simulink model "TestBenchModel"  (R2019b)
settings: Solver=VariableStepAuto  StartTime=0.0  StopTime=60  FixedStep=0.0001  RelTol=1e-3  EnableMultiTasking=on
InitFcn:
  | TestBenchData;
StartFcn:
  | TestBenchData;
values from neighbouring files (symbols this model uses):
  C = 0.0056    [TestBenchData.m]
  C1 = C    (= 0.0056)    [TestBenchData.m]
  C2 = C1    (= 0.0056)    [TestBenchData.m]
  C3 = C1    (= 0.0056)    [TestBenchData.m]
  C4 = C1    (= 0.0056)    [TestBenchData.m]
  C5 = C1    (= 0.0056)    [TestBenchData.m]
  C6 = C1    (= 0.0056)    [TestBenchData.m]
  Cfc = 0.35    [TestBenchData.m]
  Fs = 1000    [TestBenchData.m]
  glg = 4    [TestBenchData.m]
  gug = 3    [TestBenchData.m]
  Ic1 = 0.05*10^(-3)    (= 5e-05)    [TestBenchData.m]
  Ic4 = Ic3    (= 0.00012)    [TestBenchData.m]
  Ic_mf = 1.1420e-04    (= 0.0001142)    [TestBenchData.m]
  Ifc_1 = 0.003*10^(-3)    (= 3e-06)    [TestBenchData.m]
  Ifc_2 = 0.003*10^(-3)    (= 3e-06)    [TestBenchData.m]
  Imotor = 0.00068    [TestBenchData.m]
  Iprop = gml^2*I_ML + I_GL + Iprop0    [TestBenchData.m]
  Kc1 = 41.9*10^3    (= 41900)    [TestBenchData.m]
  Kc2 = Kc1    (= 41900)    [TestBenchData.m]
  Kc3 = 31*10^3    (= 31000)    [TestBenchData.m]
  Kc4 = Kc3    (= 31000)    [TestBenchData.m]
  Kc5 = 138*10^3    (= 138000)    [TestBenchData.m]
  Kc6 = Kc5    (= 138000)    [TestBenchData.m]
  Kc_mf = 1.9039e+05    (= 190390)    [TestBenchData.m]
  Kfc = 90    [TestBenchData.m]
  Klg = 44.3*10^3    (= 44300)    [TestBenchData.m]
  Km1 = 5.4*10^3    (= 5400)    [TestBenchData.m]
  Km2 = 20*10^3    (= 20000)    [TestBenchData.m]
  Kug = 43.3*10^3    (= 43300)    [TestBenchData.m]
  lg = C1    (= 0.0056)    [TestBenchData.m]
  M1 = S1    (= 0.0056)    [TestBenchData.m]
  M2 = M1    (= 0.0056)    [TestBenchData.m]
  n = 3221    [TestBenchData.m]
  n_idle = 0    [TestBenchData.m]
  Nmill = 12    [TestBenchData.m]
  P = 1150    [TestBenchData.m]
  prop_blades = 4    [TestBenchData.m]
  S = 0.0056    [TestBenchData.m]
  S1 = S    (= 0.0056)    [TestBenchData.m]
  S2 = S1    (= 0.0056)    [TestBenchData.m]
  S3 = S1    (= 0.0056)    [TestBenchData.m]
  S4 = S1    (= 0.0056)    [TestBenchData.m]
  S5 = S1    (= 0.0056)    [TestBenchData.m]
  T = P/(n/9.55)    (= 3.40965538653)    [TestBenchData.m]
  Tice = 100000    [TestBenchData.m]
  To = 0.2    [TestBenchData.m]
  Todelta = 0.5    [TestBenchData.m]
  ug = C1    (= 0.0056)    [TestBenchData.m]
  W = 131.9469    [TestBenchData.m]
  x4 = 0.06/4    (= 0.015)    [TestBenchData.m]
  x8 = 0.02/4    (= 0.005)    [TestBenchData.m]
  Z = 4    [TestBenchData.m]
  z1 = 17    [TestBenchData.m]
  z2 = 42    [TestBenchData.m]
undefined symbols (not defined in the file or in its folder): C1_22, C1_3, C_crank, C_cyl, Data, Iem, Is1, Is2, Is3, Is4, Is5, K1_11, K1_13, K1_15, K1_21, K1_23, K1_5, K1_7, K1_9, Ks1, Ks2, Ks3, Ks4, Ks5, Ks_mf, RPM, Tu
libraries: fl_lib x201, nesl_utility x92, simulink x22, dspstat3 x1
(part 1 of 3)
settings Model: Creator=jupo  LastModifiedBy=Mikael
settings DataIOCC: LimitDataPoints=on  SaveFormat=Array  SignalLoggingSaveFormat=ModelDataLogs  ReturnWorkspaceOutputs=off
settings OptimizationCC: BlockReduction=off  DefaultParameterBehavior=Inlined  BufferReuse=off  ExpressionDepthLimit=2147483647  LifeSpan=inf
settings DebuggingCC: UnderspecifiedInitializationDetection=Classic  MergeDetectMultiDrivingBlocksExec=none  SolverPrmCheckMsg=warning  FcnCallInpInsideContextMsg=warning  StateNameClashWarn=warning  SFUnexpectedBacktrackingDiag=warning  SFNoUnconditionalDefaultTransitionDiag=warning  ArithmeticOperatorsInVariantConditions=warning
settings HardwareCC: ProdBitPerPointer=32  ProdBitPerSizeT=32  ProdBitPerPtrDiffT=32  ProdLargestAtomicFloat=None  ProdWordSize=32  ProdHWDeviceType=Intel->x86/Pentium
settings ModelReferenceCC: EnableParallelModelReferenceBuilds=on  PropagateSignalLabelsOutOfModel=off
settings SFSimCC: SimUseLocalCustomCode=off  CustomCodeUndefinedFunction=UseInterfaceOnly
settings RTWCC: RTWUseLocalCustomCode=off
settings CodeAppCC: StateflowObjectComments=on
settings GRTTargetCC: TargetLangStandard=C89/C90 (ANSI)  GeneratePreprocessorConditionals=Disable all  CombineOutputUpdateFcns=off  GRTInterface=on
settings ConfigComp: CovMetricSettings=dw  CovHtmlReporting=on  CovSaveCumulativeToWorkspaceVar=on  CovSaveSingleToWorkspaceVar=on  CovExternalEMLEnable=off
settings SimscapeCC: SimscapeNormalizeSystem=off

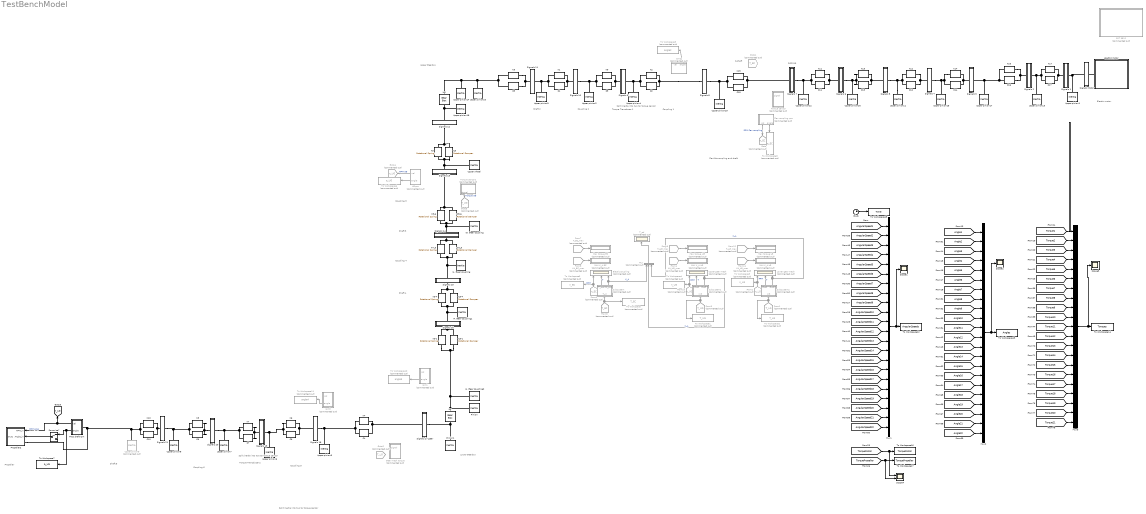
== system TestBenchModel ==
  note: Split inertia into two tor torque sensor
  note: Upper
      | Gearbox
  note: Torque Transducer 1
  note: Coupling 2
  note: Flexible coupling and shaft
  note: Electric motor
  note: Coupling 1
  note: Coupling 3
  note: Coupling 4
  note: Shaft 3
  note: Lower
      | Gearbox
  note: Shaft 4
  note: Shaft 2
  note: Coupling 5
  note: Torque
      | Transducer 2
  note: Shaft 5
  note: Coupling 6
  note: DS2315
  note: C-shaft
  note: Propeller
  note: Split inertia into two tor torque sensor
  note: Split inertia into two tor torque sensor
  C1 : fl_lib/Mechanical/Rotational Elements/Rotational Damper  D=C2*Kc2/W N*m/(rad/s)  w_specify=off  w_priority=None  w=0 rad/s  w_nominal_specify=off  w_nominal_unit=rad/s  w_nominal_value=1  t_specify=off  t_priority=None  t=0 N*m  t_nominal_specify=off  t_nominal_unit=N*m  t_nominal_value=1
      settings: AttributesFormatString=%<D>
  C10 : fl_lib/Mechanical/Rotational Elements/Rotational Damper  D=S5*Ks5/W N*m/(rad/s)  w_specify=off  w_priority=None  w=0 rad/s  w_nominal_specify=off  w_nominal_unit=rad/s  w_nominal_value=1  t_specify=off  t_priority=None  t=0 N*m  t_nominal_specify=off  t_nominal_unit=N*m  t_nominal_value=1
      settings: AttributesFormatString=%<D>
  C{11..14} (4 alike) : fl_lib/Mechanical/Rotational Elements/Rotational Damper  D=Cfc*Kfc/W N*m/(rad/s)  w_specify=off  w_priority=None  w=0 rad/s  w_nominal_specify=off  w_nominal_unit=rad/s  w_nominal_value=1  t_specify=off  t_priority=None  t=0 N*m  t_nominal_specify=off  t_nominal_unit=N*m  t_nominal_value=1
      settings: AttributesFormatString=%<D>
  C15 : fl_lib/Mechanical/Rotational Elements/Rotational Damper  D=S1*Ks1/W N*m/(rad/s)  w_specify=off  w_priority=None  w=0 rad/s  w_nominal_specify=off  w_nominal_unit=rad/s  w_nominal_value=1  t_specify=off  t_priority=None  t=0 N*m  t_nominal_specify=off  t_nominal_unit=N*m  t_nominal_value=1
      settings: AttributesFormatString=%<D>
  C16 : fl_lib/Mechanical/Rotational Elements/Rotational Damper  D=S*Ks_mf/W N*m/(rad/s)  w_specify=off  w_priority=None  w=0 rad/s  w_nominal_specify=off  w_nominal_unit=rad/s  w_nominal_value=1  t_specify=off  t_priority=None  t=0 N*m  t_nominal_specify=off  t_nominal_unit=N*m  t_nominal_value=1
      settings: AttributesFormatString=%<D>
  C17 : fl_lib/Mechanical/Rotational Elements/Rotational Damper  D=C*Kc_mf/W N*m/(rad/s)  w_specify=off  w_priority=None  w=0 rad/s  w_nominal_specify=off  w_nominal_unit=rad/s  w_nominal_value=1  t_specify=off  t_priority=None  t=0 N*m  t_nominal_specify=off  t_nominal_unit=N*m  t_nominal_value=1
      settings: AttributesFormatString=%<D>
  C2 : fl_lib/Mechanical/Rotational Elements/Rotational Damper  D=C1*Kc1/W N*m/(rad/s)  w_specify=off  w_priority=None  w=0 rad/s  w_nominal_specify=off  w_nominal_unit=rad/s  w_nominal_value=1  t_specify=off  t_priority=None  t=0 N*m  t_nominal_specify=off  t_nominal_unit=N*m  t_nominal_value=1
      settings: AttributesFormatString=%<D>
  C3 : fl_lib/Mechanical/Rotational Elements/Rotational Damper  D=ug*Kug/W N*m/(rad/s)  w_specify=off  w_priority=None  w=0 rad/s  w_nominal_specify=off  w_nominal_unit=rad/s  w_nominal_value=1  t_specify=off  t_priority=None  t=0 N*m  t_nominal_specify=off  t_nominal_unit=N*m  t_nominal_value=1
      settings: AttributesFormatString=%<D>
  C3-1 : fl_lib/Mechanical/Rotational Elements/Rotational Damper  D=S4*Ks4/W N*m/(rad/s)  w_specify=off  w_priority=None  w=0 rad/s  w_nominal_specify=off  w_nominal_unit=rad/s  w_nominal_value=1  t_specify=off  t_priority=None  t=0 N*m  t_nominal_specify=off  t_nominal_unit=N*m  t_nominal_value=1
      settings: AttributesFormatString=%<D>
  C3-4 : fl_lib/Mechanical/Rotational Elements/Rotational Damper  D=C4*Kc4/W N*m/(rad/s)  w_specify=off  w_priority=None  w=0 rad/s  w_nominal_specify=off  w_nominal_unit=rad/s  w_nominal_value=1  t_specify=off  t_priority=None  t=0 N*m  t_nominal_specify=off  t_nominal_unit=N*m  t_nominal_value=1
      settings: AttributesFormatString=%<D>
  C4 : fl_lib/Mechanical/Rotational Elements/Rotational Damper  D=lg*Klg/W N*m/(rad/s)  w_specify=off  w_priority=None  w=0 rad/s  w_nominal_specify=off  w_nominal_unit=rad/s  w_nominal_value=1  t_specify=off  t_priority=None  t=0 N*m  t_nominal_specify=off  t_nominal_unit=N*m  t_nominal_value=1
      settings: AttributesFormatString=%<D>
  C4_5 : fl_lib/Mechanical/Rotational Elements/Rotational Damper  D=S3*Ks3/W N*m/(rad/s)  w_specify=off  w_priority=None  w=0 rad/s  w_nominal_specify=off  w_nominal_unit=rad/s  w_nominal_value=1  t_specify=off  t_priority=None  t=0 N*m  t_nominal_specify=off  t_nominal_unit=N*m  t_nominal_value=1
      settings: AttributesFormatString=%<D>
  C5 : fl_lib/Mechanical/Rotational Elements/Rotational Damper  D=S2*Ks2/W N*m/(rad/s)  w_specify=off  w_priority=None  w=0 rad/s  w_nominal_specify=off  w_nominal_unit=rad/s  w_nominal_value=1  t_specify=off  t_priority=None  t=0 N*m  t_nominal_specify=off  t_nominal_unit=N*m  t_nominal_value=1
      settings: AttributesFormatString=%<D>
  C5-6 : fl_lib/Mechanical/Rotational Elements/Rotational Damper  D=C3*Kc3/W N*m/(rad/s)  w_specify=off  w_priority=None  w=0 rad/s  w_nominal_specify=off  w_nominal_unit=rad/s  w_nominal_value=1  t_specify=off  t_priority=None  t=0 N*m  t_nominal_specify=off  t_nominal_unit=N*m  t_nominal_value=1
      settings: AttributesFormatString=%<D>
  C6 : fl_lib/Mechanical/Rotational Elements/Rotational Damper  D=C5*Kc5/W N*m/(rad/s)  w_specify=off  w_priority=None  w=0 rad/s  w_nominal_specify=off  w_nominal_unit=rad/s  w_nominal_value=1  t_specify=off  t_priority=None  t=0 N*m  t_nominal_specify=off  t_nominal_unit=N*m  t_nominal_value=1
      settings: AttributesFormatString=%<D>
  C7 : fl_lib/Mechanical/Rotational Elements/Rotational Damper  D=M2*Km2/W N*m/(rad/s)  w_specify=off  w_priority=None  w=0 rad/s  w_nominal_specify=off  w_nominal_unit=rad/s  w_nominal_value=1  t_specify=off  t_priority=None  t=0 N*m  t_nominal_specify=off  t_nominal_unit=N*m  t_nominal_value=1
      settings: AttributesFormatString=%<D>
  C8 : fl_lib/Mechanical/Rotational Elements/Rotational Damper  D=C6*Kc6/W N*m/(rad/s)  w_specify=off  w_priority=None  w=0 rad/s  w_nominal_specify=off  w_nominal_unit=rad/s  w_nominal_value=1  t_specify=off  t_priority=None  t=0 N*m  t_nominal_specify=off  t_nominal_unit=N*m  t_nominal_value=1
      settings: AttributesFormatString=%<D>
  C9 : fl_lib/Mechanical/Rotational Elements/Rotational Damper  D=M1*Km1/W N*m/(rad/s)  w_specify=off  w_priority=None  w=0 rad/s  w_nominal_specify=off  w_nominal_unit=rad/s  w_nominal_value=1  t_specify=off  t_priority=None  t=0 N*m  t_nominal_specify=off  t_nominal_unit=N*m  t_nominal_value=1
      settings: AttributesFormatString=%<D>
  CAT 3512 : Subsystem  Commented=on
      mask Display: image(imread('3512B.jpg'))
  Clock : Clock
  Elastic coupling : Scope  Commented=on  NumInputPorts=3
  Flex coupling rpm : Subsystem  Commented=on
  From1 : From  Commented=on  GotoTag=T_LG  TagVisibility=global
  From10 : From  Commented=on  GotoTag=n_UG  TagVisibility=global
  From11 : From  Commented=on  GotoTag=KA_LG_max  TagVisibility=global
  From12 : From  Commented=on  GotoTag=T_LG_max  TagVisibility=global
  From2 : From  Commented=on  GotoTag=n_LG  TagVisibility=global
  From3 : From  Commented=on  GotoTag=T_UG  TagVisibility=global
  From4 : From  Commented=on  GotoTag=KA_UG_max  TagVisibility=global
  From5 : From  Commented=on  GotoTag=T_EC  TagVisibility=global
  From6 : From  Commented=on  GotoTag=n_EC  TagVisibility=global
  From7 : From  Commented=on  GotoTag=T_EC_max  TagVisibility=global
  From8 : From  Commented=on  GotoTag=KA_EC_max  TagVisibility=global
  From9 : From  Commented=on  GotoTag=T_UG_max  TagVisibility=global
  Gear mesh torque : Subsystem  Commented=on
  Goto : Goto  Commented=on  GotoTag=n_EC  TagVisibility=global
  Goto1 : Goto  Commented=on  GotoTag=T_EC  TagVisibility=global
  Goto2 : Goto  Commented=on  GotoTag=T_LG  TagVisibility=global
  Goto4 : Goto  Commented=on  GotoTag=n_UG  TagVisibility=global
  Goto5 : Goto  Commented=on  GotoTag=T_UG  TagVisibility=global
  "I4, Gear coupling" : fl_lib/Mechanical/Rotational Elements/Inertia  inertia=Ic4 + Is3/2 kg*m^2  w_specify=off  w_priority=High  w=-n_idle*(z1/z2) rpm  w_nominal_specify=off  w_nominal_unit=rad/s  w_nominal_value=1  t_specify=off  t_priority=None  t=0 N*m  t_nominal_specify=off  t_nominal_unit=N*m  t_nominal_value=1
      settings: AttributesFormatString=%<inertia>
  "I4, Gear coupling1" : fl_lib/Mechanical/Rotational Elements/Inertia  inertia=Is4/2 kg*m^2  w_specify=off  w_priority=High  w=-n_idle*(z1/z2) rpm  w_nominal_specify=off  w_nominal_unit=rad/s  w_nominal_value=1  t_specify=off  t_priority=None  t=0 N*m  t_nominal_specify=off  t_nominal_unit=N*m  t_nominal_value=1
      settings: AttributesFormatString=%<inertia>
  "I4, Gear coupling2" : fl_lib/Mechanical/Rotational Elements/Inertia  inertia=Is4/2 kg*m^2  w_specify=off  w_priority=High  w=-n_idle*(z1/z2) rpm  w_nominal_specify=off  w_nominal_unit=rad/s  w_nominal_value=1  t_specify=off  t_priority=None  t=0 N*m  t_nominal_specify=off  t_nominal_unit=N*m  t_nominal_value=1
      settings: AttributesFormatString=%<inertia>
  "I5, Gear coupling" : fl_lib/Mechanical/Rotational Elements/Inertia  inertia=Is3/2 kg*m^2  w_specify=off  w_priority=High  w=-n_idle*(z1/z2) rpm  w_nominal_specify=off  w_nominal_unit=rad/s  w_nominal_value=1  t_specify=off  t_priority=None  t=0 N*m  t_nominal_specify=off  t_nominal_unit=N*m  t_nominal_value=1
      settings: AttributesFormatString=%<inertia>
  K1 : fl_lib/Mechanical/Rotational Elements/Rotational Spring  spr_rate=Kc2 N*m/rad  w_specify=off  w_priority=None  w=0 rad/s  w_nominal_specify=off  w_nominal_unit=rad/s  w_nominal_value=1  t_specify=off  t_priority=None  t=0 N*m  t_nominal_specify=off  t_nominal_unit=N*m  t_nominal_value=1  phi_specify=on  phi_priority=High  phi=0 rad  phi_nominal_specify=off  phi_nominal_unit=rad  phi_nominal_value=1
      settings: AttributesFormatString=%<spr_rate>  SourceProductName=Simscape
  K10 : fl_lib/Mechanical/Rotational Elements/Rotational Spring  spr_rate=Ks5 N*m/rad  w_specify=off  w_priority=None  w=0 rad/s  w_nominal_specify=off  w_nominal_unit=rad/s  w_nominal_value=1  t_specify=off  t_priority=None  t=0 N*m  t_nominal_specify=off  t_nominal_unit=N*m  t_nominal_value=1  phi_specify=on  phi_priority=High  phi=0 rad  phi_nominal_specify=off  phi_nominal_unit=rad  phi_nominal_value=1
      settings: AttributesFormatString=%<spr_rate>  SourceProductName=Simscape
  K{11..14} (4 alike) : fl_lib/Mechanical/Rotational Elements/Rotational Spring  spr_rate=Kfc N*m/rad  w_specify=off  w_priority=None  w=0 rad/s  w_nominal_specify=off  w_nominal_unit=rad/s  w_nominal_value=1  t_specify=off  t_priority=None  t=0 N*m  t_nominal_specify=off  t_nominal_unit=N*m  t_nominal_value=1  phi_specify=on  phi_priority=High  phi=0 rad  phi_nominal_specify=off  phi_nominal_unit=rad  phi_nominal_value=1
      settings: AttributesFormatString=%<spr_rate>  SourceProductName=Simscape
  K15 : fl_lib/Mechanical/Rotational Elements/Rotational Spring  spr_rate=Ks1 N*m/rad  w_specify=off  w_priority=None  w=0 rad/s  w_nominal_specify=off  w_nominal_unit=rad/s  w_nominal_value=1  t_specify=off  t_priority=None  t=0 N*m  t_nominal_specify=off  t_nominal_unit=N*m  t_nominal_value=1  phi_specify=on  phi_priority=High  phi=0 rad  phi_nominal_specify=off  phi_nominal_unit=rad  phi_nominal_value=1
      settings: AttributesFormatString=%<spr_rate>  SourceProductName=Simscape
  K16 : fl_lib/Mechanical/Rotational Elements/Rotational Spring  spr_rate=Ks_mf N*m/rad  w_specify=off  w_priority=None  w=0 rad/s  w_nominal_specify=off  w_nominal_unit=rad/s  w_nominal_value=1  t_specify=off  t_priority=None  t=0 N*m  t_nominal_specify=off  t_nominal_unit=N*m  t_nominal_value=1  phi_specify=on  phi_priority=High  phi=0 rad  phi_nominal_specify=off  phi_nominal_unit=rad  phi_nominal_value=1
      settings: AttributesFormatString=%<spr_rate>  SourceProductName=Simscape
  K17 : fl_lib/Mechanical/Rotational Elements/Rotational Spring  spr_rate=Kc_mf N*m/rad  w_specify=off  w_priority=None  w=0 rad/s  w_nominal_specify=off  w_nominal_unit=rad/s  w_nominal_value=1  t_specify=off  t_priority=None  t=0 N*m  t_nominal_specify=off  t_nominal_unit=N*m  t_nominal_value=1  phi_specify=on  phi_priority=High  phi=0 rad  phi_nominal_specify=off  phi_nominal_unit=rad  phi_nominal_value=1
      settings: AttributesFormatString=%<spr_rate>  SourceProductName=Simscape
  K2 : fl_lib/Mechanical/Rotational Elements/Rotational Spring  spr_rate=Kc1 N*m/rad  w_specify=off  w_priority=None  w=0 rad/s  w_nominal_specify=off  w_nominal_unit=rad/s  w_nominal_value=1  t_specify=off  t_priority=None  t=0 N*m  t_nominal_specify=off  t_nominal_unit=N*m  t_nominal_value=1  phi_specify=on  phi_priority=High  phi=0 rad  phi_nominal_specify=off  phi_nominal_unit=rad  phi_nominal_value=1
      settings: AttributesFormatString=%<spr_rate>  SourceProductName=Simscape
  K3 : fl_lib/Mechanical/Rotational Elements/Rotational Spring  spr_rate=Kug N*m/rad  w_specify=off  w_priority=None  w=0 rad/s  w_nominal_specify=off  w_nominal_unit=rad/s  w_nominal_value=1  t_specify=off  t_priority=None  t=0 N*m  t_nominal_specify=off  t_nominal_unit=N*m  t_nominal_value=1  phi_specify=on  phi_priority=High  phi=0 rad  phi_nominal_specify=off  phi_nominal_unit=rad  phi_nominal_value=1
      settings: AttributesFormatString=%<spr_rate>  SourceProductName=Simscape
  K3-1 : fl_lib/Mechanical/Rotational Elements/Rotational Spring  spr_rate=Ks4 N*m/rad  w_specify=off  w_priority=None  w=0 rad/s  w_nominal_specify=off  w_nominal_unit=rad/s  w_nominal_value=1  t_specify=off  t_priority=None  t=0 N*m  t_nominal_specify=off  t_nominal_unit=N*m  t_nominal_value=1  phi_specify=on  phi_priority=High  phi=0 rad  phi_nominal_specify=off  phi_nominal_unit=rad  phi_nominal_value=1
      settings: AttributesFormatString=%<spr_rate>  SourceProductName=Simscape
  K3-4 : fl_lib/Mechanical/Rotational Elements/Rotational Spring  spr_rate=Kc4 N*m/rad  w_specify=off  w_priority=None  w=0 rad/s  w_nominal_specify=off  w_nominal_unit=rad/s  w_nominal_value=1  t_specify=off  t_priority=None  t=0 N*m  t_nominal_specify=off  t_nominal_unit=N*m  t_nominal_value=1  phi_specify=on  phi_priority=High  phi=0 rad  phi_nominal_specify=off  phi_nominal_unit=rad  phi_nominal_value=1
      settings: AttributesFormatString=%<spr_rate>  SourceProductName=Simscape
  K4 : fl_lib/Mechanical/Rotational Elements/Rotational Spring  spr_rate=Klg N*m/rad  w_specify=off  w_priority=None  w=0 rad/s  w_nominal_specify=off  w_nominal_unit=rad/s  w_nominal_value=1  t_specify=off  t_priority=None  t=0 N*m  t_nominal_specify=off  t_nominal_unit=N*m  t_nominal_value=1  phi_specify=on  phi_priority=High  phi=0 rad  phi_nominal_specify=off  phi_nominal_unit=rad  phi_nominal_value=1
      settings: AttributesFormatString=%<spr_rate>  SourceProductName=Simscape
  K4_5 : fl_lib/Mechanical/Rotational Elements/Rotational Spring  spr_rate=Ks3 N*m/rad  w_specify=off  w_priority=None  w=0 rad/s  w_nominal_specify=off  w_nominal_unit=rad/s  w_nominal_value=1  t_specify=off  t_priority=None  t=0 N*m  t_nominal_specify=off  t_nominal_unit=N*m  t_nominal_value=1  phi_specify=on  phi_priority=High  phi=0 rad  phi_nominal_specify=off  phi_nominal_unit=rad  phi_nominal_value=1
      settings: AttributesFormatString=%<spr_rate>  SourceProductName=Simscape
  K5 : fl_lib/Mechanical/Rotational Elements/Rotational Spring  spr_rate=Ks2 N*m/rad  w_specify=off  w_priority=None  w=0 rad/s  w_nominal_specify=off  w_nominal_unit=rad/s  w_nominal_value=1  t_specify=off  t_priority=None  t=0 N*m  t_nominal_specify=off  t_nominal_unit=N*m  t_nominal_value=1  phi_specify=on  phi_priority=High  phi=0 rad  phi_nominal_specify=off  phi_nominal_unit=rad  phi_nominal_value=1
      settings: AttributesFormatString=%<spr_rate>  SourceProductName=Simscape
  K5-6 : fl_lib/Mechanical/Rotational Elements/Rotational Spring  spr_rate=Kc3 N*m/rad  w_specify=off  w_priority=None  w=0 rad/s  w_nominal_specify=off  w_nominal_unit=rad/s  w_nominal_value=1  t_specify=off  t_priority=None  t=0 N*m  t_nominal_specify=off  t_nominal_unit=N*m  t_nominal_value=1  phi_specify=on  phi_priority=High  phi=0 rad  phi_nominal_specify=off  phi_nominal_unit=rad  phi_nominal_value=1
      settings: AttributesFormatString=%<spr_rate>  SourceProductName=Simscape
  K6 : fl_lib/Mechanical/Rotational Elements/Rotational Spring  spr_rate=Kc5 N*m/rad  w_specify=off  w_priority=None  w=0 rad/s  w_nominal_specify=off  w_nominal_unit=rad/s  w_nominal_value=1  t_specify=off  t_priority=None  t=0 N*m  t_nominal_specify=off  t_nominal_unit=N*m  t_nominal_value=1  phi_specify=on  phi_priority=High  phi=0 rad  phi_nominal_specify=off  phi_nominal_unit=rad  phi_nominal_value=1
      settings: AttributesFormatString=%<spr_rate>  SourceProductName=Simscape
  K7 : fl_lib/Mechanical/Rotational Elements/Rotational Spring  spr_rate=Km2 N*m/rad  w_specify=off  w_priority=None  w=0 rad/s  w_nominal_specify=off  w_nominal_unit=rad/s  w_nominal_value=1  t_specify=off  t_priority=None  t=0 N*m  t_nominal_specify=off  t_nominal_unit=N*m  t_nominal_value=1  phi_specify=on  phi_priority=High  phi=0 rad  phi_nominal_specify=off  phi_nominal_unit=rad  phi_nominal_value=1
      settings: AttributesFormatString=%<spr_rate>  SourceProductName=Simscape
  K8 : fl_lib/Mechanical/Rotational Elements/Rotational Spring  spr_rate=Kc6 N*m/rad  w_specify=off  w_priority=None  w=0 rad/s  w_nominal_specify=off  w_nominal_unit=rad/s  w_nominal_value=1  t_specify=off  t_priority=None  t=0 N*m  t_nominal_specify=off  t_nominal_unit=N*m  t_nominal_value=1  phi_specify=on  phi_priority=High  phi=0 rad  phi_nominal_specify=off  phi_nominal_unit=rad  phi_nominal_value=1
      settings: AttributesFormatString=%<spr_rate>  SourceProductName=Simscape
  K9 : fl_lib/Mechanical/Rotational Elements/Rotational Spring  spr_rate=Km1 N*m/rad  w_specify=off  w_priority=None  w=0 rad/s  w_nominal_specify=off  w_nominal_unit=rad/s  w_nominal_value=1  t_specify=off  t_priority=None  t=0 N*m  t_nominal_specify=off  t_nominal_unit=N*m  t_nominal_value=1  phi_specify=on  phi_priority=High  phi=0 rad  phi_nominal_specify=off  phi_nominal_unit=rad  phi_nominal_value=1
      settings: AttributesFormatString=%<spr_rate>  SourceProductName=Simscape
  LG : fl_lib/Mechanical/Mechanisms/Gear Box  ratio=glg  t_in_specify=off  t_in_priority=None  t_in=0 N*m  t_in_nominal_specify=off  t_in_nominal_unit=N*m  t_in_nominal_value=1  t_out_specify=off  t_out_priority=None  t_out=0 N*m  t_out_nominal_specify=off  t_out_nominal_unit=N*m  t_out_nominal_value=1
  Lower gear mesh : Scope  Commented=on  NumInputPorts=3
  MAX K_A EC : Display  Commented=on
  MAX K_A LG : Display  Commented=on
  MAX K_A UG : Display  Commented=on
  Max torque EC : Display  Commented=on
  Max torque LG : Display  Commented=on
  Max torque UG : Display  Commented=on
  Mux : Mux  Commented=on  Inputs=3
  Mux1 : Mux  Inputs=22
  Mux2 : Mux  Inputs=22
  Mux3 : Mux  Inputs=21
  Pinion : fl_lib/Mechanical/Rotational Elements/Inertia  inertia=I_lowerpinion kg*m^2  w_specify=off  w_priority=High  w=-n_idle*(z1/z2) rpm  w_nominal_specify=off  w_nominal_unit=rad/s  w_nominal_value=1  t_specify=off  t_priority=None  t=0 N*m  t_nominal_specify=off  t_nominal_unit=N*m  t_nominal_value=1
      settings: AttributesFormatString=%<inertia>
  Pinion1 : fl_lib/Mechanical/Rotational Elements/Inertia  inertia=I_lowerwheel kg*m^2  w_specify=off  w_priority=High  w=-n_idle*(z1/z2) rpm  w_nominal_specify=off  w_nominal_unit=rad/s  w_nominal_value=1  t_specify=off  t_priority=None  t=0 N*m  t_nominal_specify=off  t_nominal_unit=N*m  t_nominal_value=1
      settings: AttributesFormatString=%<inertia>
  Prop shaft rpm : Subsystem
  Propeller2 : Subsystem
      mask Display: image(imread('prop.png'))
  Scope1 : Scope
  Scope2 : Scope
  Scope3 : Scope
  Scope4 : Scope  NumInputPorts=2
  Signals 1 : Subsystem
  Signals 10 : Subsystem
  Signals 11 : Subsystem
  Signals 12 : Subsystem
  Signals 13 : Subsystem
  Signals 14 : Subsystem
  Signals 15 : Subsystem
  Signals 16 : Subsystem
  Signals 17 gear : Subsystem
  Signals 18 : Subsystem
  Signals 19 : Subsystem
  Signals 2 : Subsystem
  Signals 20 : Subsystem
  Signals 21 : Subsystem
  Signals 3 : Subsystem
  Signals 4 : Subsystem
  Signals 5 : Subsystem
  Signals 6 : Subsystem
  Signals 7 : Subsystem
  Signals 8 : Subsystem
  Signals 9 : Subsystem
  Signals Motor : Subsystem
  Some ice? : ManualSwitch
  Subsystem : Subsystem  Commented=on
  Subsystem1 : Subsystem  Commented=on
  Subsystem2 : Subsystem  Commented=on
  T_rel : Scope  Commented=on
  To Workspace : ToWorkspace  Commented=on  VariableName=T_EC  SaveFormat=Timeseries  SampleTime=-1
  To Workspace1 : ToWorkspace  Commented=on  VariableName=T_UG  SaveFormat=Timeseries  SampleTime=-1
  To Workspace10 : ToWorkspace  Commented=on  VariableName=angle3  SaveFormat=Timeseries  SampleTime=-1
  To Workspace11 : ToWorkspace  Commented=on  VariableName=angle4  SaveFormat=Timeseries  SampleTime=-1
  To Workspace12 : ToWorkspace  VariableName=AngularSpeeds  SampleTime=1/Fs
  To Workspace13 : ToWorkspace  VariableName=Angles  SampleTime=1/Fs
  To Workspace14 : ToWorkspace  VariableName=Torques  SampleTime=1/Fs
  To Workspace15 : ToWorkspace  VariableName=Time  SampleTime=1/Fs
  To Workspace16 : ToWorkspace  VariableName=TorqueMotor  SampleTime=1/Fs
  To Workspace17 : ToWorkspace  VariableName=TorquePropeller  SampleTime=1/Fs
  To Workspace2 : ToWorkspace  Commented=on  VariableName=T_LG  SaveFormat=Timeseries  SampleTime=-1
  To Workspace3 : ToWorkspace  Commented=on  VariableName=n_EC  SaveFormat=Timeseries  SampleTime=-1
  To Workspace4 : ToWorkspace  Commented=on  VariableName=n_UG  SaveFormat=Timeseries  SampleTime=-1
  To Workspace5 : ToWorkspace  Commented=on  VariableName=n_LG  SaveFormat=Timeseries  SampleTime=-1
  To Workspace6 : ToWorkspace  Commented=on  VariableName=a_UG  SaveFormat=Timeseries  SampleTime=-1
  To Workspace7 : ToWorkspace  VariableName=a_LG  SaveFormat=Timeseries  SampleTime=-1
  To Workspace8 : ToWorkspace  Commented=on  VariableName=a_EC  SaveFormat=Timeseries  SampleTime=-1
  To Workspace9 : ToWorkspace  Commented=on  VariableName=angle2  SaveFormat=Timeseries  SampleTime=-1
  Torque sensor : Subsystem  Commented=on
  Torque sensor1 : Subsystem  Commented=on
  UG : fl_lib/Mechanical/Mechanisms/Gear Box  ratio=gug  t_in_specify=off  t_in_priority=None  t_in=0 N*m  t_in_nominal_specify=off  t_in_nominal_unit=N*m  t_in_nominal_value=1  t_out_specify=off  t_out_priority=None  t_out=0 N*m  t_out_nominal_specify=off  t_out_nominal_unit=N*m  t_out_nominal_value=1
  UGrpm : Subsystem  Commented=on
  Upper gear mesh : Scope  Commented=on  NumInputPorts=3
  Upper pinion1 : fl_lib/Mechanical/Rotational Elements/Inertia  inertia=Ic_mf + Imotor kg*m^2  w_specify=off  w_priority=High  w=n_idle rpm  w_nominal_specify=off  w_nominal_unit=rad/s  w_nominal_value=1  t_specify=off  t_priority=None  t=0 N*m  t_nominal_specify=off  t_nominal_unit=N*m  t_nominal_value=1
      settings: AttributesFormatString=%<inertia>
  Upper pinion10 : fl_lib/Mechanical/Rotational Elements/Inertia  inertia=Is2/2 kg*m^2  w_specify=on  w_priority=High  w=n_idle rpm  w_nominal_specify=off  w_nominal_unit=rad/s  w_nominal_value=1  t_specify=off  t_priority=None  t=0 N*m  t_nominal_specify=off  t_nominal_unit=N*m  t_nominal_value=1
      settings: AttributesFormatString=%<inertia>
  Upper pinion11 : fl_lib/Mechanical/Rotational Elements/Inertia  inertia=Ifc_2 + Iem + Ifc_1 kg*m^2  w_specify=on  w_priority=High  w=n_idle rpm  w_nominal_specify=off  w_nominal_unit=rad/s  w_nominal_value=1  t_specify=off  t_priority=None  t=0 N*m  t_nominal_specify=off  t_nominal_unit=N*m  t_nominal_value=1
      settings: AttributesFormatString=%<inertia>
  Upper pinion12 : fl_lib/Mechanical/Rotational Elements/Inertia  inertia=Ifc_2 + Is1/2 kg*m^2  w_specify=on  w_priority=High  w=n_idle rpm  w_nominal_specify=off  w_nominal_unit=rad/s  w_nominal_value=1  t_specify=off  t_priority=None  t=0 N*m  t_nominal_specify=off  t_nominal_unit=N*m  t_nominal_value=1
      settings: AttributesFormatString=%<inertia>
  Upper pinion13 : fl_lib/Mechanical/Rotational Elements/Inertia  inertia=Is_mf kg*m^2  w_specify=off  w_priority=High  w=n_idle rpm  w_nominal_specify=off  w_nominal_unit=rad/s  w_nominal_value=1  t_specify=off  t_priority=None  t=0 N*m  t_nominal_specify=off  t_nominal_unit=N*m  t_nominal_value=1
      settings: AttributesFormatString=%<inertia>
  Upper pinion14 : fl_lib/Mechanical/Rotational Elements/Inertia  inertia=I_upperpinion kg*m^2  w_specify=on  w_priority=High  w=n_idle rpm  w_nominal_specify=off  w_nominal_unit=rad/s  w_nominal_value=1  t_specify=off  t_priority=None  t=0 N*m  t_nominal_specify=off  t_nominal_unit=N*m  t_nominal_value=1
      settings: AttributesFormatString=%<inertia>
  Upper pinion15 : fl_lib/Mechanical/Rotational Elements/Inertia  inertia=Ifcm kg*m^2  w_specify=on  w_priority=High  w=n_idle rpm  w_nominal_specify=off  w_nominal_unit=rad/s  w_nominal_value=1  t_specify=off  t_priority=None  t=0 N*m  t_nominal_specify=off  t_nominal_unit=N*m  t_nominal_value=1
      settings: AttributesFormatString=%<inertia>
  Upper pinion16 : fl_lib/Mechanical/Rotational Elements/Inertia  inertia=Ifcm kg*m^2  w_specify=on  w_priority=High  w=n_idle rpm  w_nominal_specify=off  w_nominal_unit=rad/s  w_nominal_value=1  t_specify=off  t_priority=None  t=0 N*m  t_nominal_specify=off  t_nominal_unit=N*m  t_nominal_value=1
      settings: AttributesFormatString=%<inertia>
  Upper pinion17 : fl_lib/Mechanical/Rotational Elements/Inertia  inertia=Ifc_1 kg*m^2  w_specify=on  w_priority=High  w=n_idle rpm  w_nominal_specify=off  w_nominal_unit=rad/s  w_nominal_value=1  t_specify=off  t_priority=None  t=0 N*m  t_nominal_specify=off  t_nominal_unit=N*m  t_nominal_value=1
      settings: AttributesFormatString=%<inertia>
  Upper pinion18 : fl_lib/Mechanical/Rotational Elements/Inertia  inertia=I_upperwheel kg*m^2  w_specify=on  w_priority=High  w=n_idle rpm  w_nominal_specify=off  w_nominal_unit=rad/s  w_nominal_value=1  t_specify=off  t_priority=None  t=0 N*m  t_nominal_specify=off  t_nominal_unit=N*m  t_nominal_value=1
      settings: AttributesFormatString=%<inertia>
  Upper pinion19 : fl_lib/Mechanical/Rotational Elements/Inertia  inertia=Is1/2 + Ic1 kg*m^2  w_specify=on  w_priority=High  w=n_idle rpm  w_nominal_specify=off  w_nominal_unit=rad/s  w_nominal_value=1  t_specify=off  t_priority=None  t=0 N*m  t_nominal_specify=off  t_nominal_unit=N*m  t_nominal_value=1
      settings: AttributesFormatString=%<inertia>
  Upper pinion2 : fl_lib/Mechanical/Rotational Elements/Inertia  inertia=Ic2 kg*m^2  w_specify=on  w_priority=High  w=n_idle rpm  w_nominal_specify=off  w_nominal_unit=rad/s  w_nominal_value=1  t_specify=off  t_priority=None  t=0 N*m  t_nominal_specify=off  t_nominal_unit=N*m  t_nominal_value=1
      settings: AttributesFormatString=%<inertia>
  Upper pinion3 : fl_lib/Mechanical/Rotational Elements/Inertia  inertia=Is2/2 kg*m^2  w_specify=on  w_priority=High  w=n_idle rpm  w_nominal_specify=off  w_nominal_unit=rad/s  w_nominal_value=1  t_specify=off  t_priority=None  t=0 N*m  t_nominal_specify=off  t_nominal_unit=N*m  t_nominal_value=1
      settings: AttributesFormatString=%<inertia>
  Upper pinion4 : fl_lib/Mechanical/Rotational Elements/Inertia  inertia=Im1 kg*m^2  w_specify=on  w_priority=High  w=n_idle rpm  w_nominal_specify=off  w_nominal_unit=rad/s  w_nominal_value=1  t_specify=off  t_priority=None  t=0 N*m  t_nominal_specify=off  t_nominal_unit=N*m  t_nominal_value=1
      settings: AttributesFormatString=%<inertia>
  Upper pinion5 : fl_lib/Mechanical/Rotational Elements/Inertia  inertia=Ic5 kg*m^2  w_specify=on  w_priority=High  w=n_idle rpm  w_nominal_specify=off  w_nominal_unit=rad/s  w_nominal_value=1  t_specify=off  t_priority=None  t=0 N*m  t_nominal_specify=off  t_nominal_unit=N*m  t_nominal_value=1
      settings: AttributesFormatString=%<inertia>
  Upper pinion6 : fl_lib/Mechanical/Rotational Elements/Inertia  inertia=Im2 kg*m^2  w_specify=on  w_priority=High  w=n_idle rpm  w_nominal_specify=off  w_nominal_unit=rad/s  w_nominal_value=1  t_specify=off  t_priority=None  t=0 N*m  t_nominal_specify=off  t_nominal_unit=N*m  t_nominal_value=1
      settings: AttributesFormatString=%<inertia>
  Upper pinion7 : fl_lib/Mechanical/Rotational Elements/Inertia  inertia=Ic6 kg*m^2  w_specify=on  w_priority=High  w=n_idle rpm  w_nominal_specify=off  w_nominal_unit=rad/s  w_nominal_value=1  t_specify=off  t_priority=None  t=0 N*m  t_nominal_specify=off  t_nominal_unit=N*m  t_nominal_value=1
      settings: AttributesFormatString=%<inertia>
  Upper pinion8 : fl_lib/Mechanical/Rotational Elements/Inertia  inertia=Is5/2 kg*m^2  w_specify=on  w_priority=High  w=n_idle rpm  w_nominal_specify=off  w_nominal_unit=rad/s  w_nominal_value=1  t_specify=off  t_priority=None  t=0 N*m  t_nominal_specify=off  t_nominal_unit=N*m  t_nominal_value=1
      settings: AttributesFormatString=%<inertia>
  Upper pinion9 : fl_lib/Mechanical/Rotational Elements/Inertia  Commented=on  inertia=Is5/2 kg*m^2  w_specify=on  w_priority=High  w=n_idle rpm  w_nominal_specify=off  w_nominal_unit=rad/s  w_nominal_value=1  t_specify=off  t_priority=None  t=0 N*m  t_nominal_specify=off  t_nominal_unit=N*m  t_nominal_value=1
      settings: AttributesFormatString=%<inertia>
  Upper wheel : fl_lib/Mechanical/Rotational Elements/Inertia  inertia=Ic3 kg*m^2  w_specify=off  w_priority=High  w=-n_idle*(z1/z2) rpm  w_nominal_specify=off  w_nominal_unit=rad/s  w_nominal_value=1  t_specify=off  t_priority=None  t=0 N*m  t_nominal_specify=off  t_nominal_unit=N*m  t_nominal_value=1
      settings: AttributesFormatString=%<inertia>
  electric motor : Subsystem
      mask Display: image(imread('e_motor.jpg'))
  rpm1 : Subsystem  Commented=on
  rpm2 : Subsystem  Commented=on
  rpm3 : Subsystem  Commented=on
  tag scope: n_LG=global
  wires:
  Prop shaft rpm/1(vel) -> Propeller2/1(RPM_in), [n_LG]  "RPM prop"
  Prop shaft rpm/2(angle) -> To Workspace7/1, Some ice?/1
  Some ice?/1 -> Propeller2/2(Angle_in)
  Subsystem/1(T_out) -> Elastic coupling/2  "T"
  Subsystem/2(KA_out) -> Elastic coupling/3, Mux/1  "K_A"
  From6/1 -> Elastic coupling/1, To Workspace3/1  "RPM"
  Subsystem2/1(Out1) -> Lower gear mesh/2  "T"
  Subsystem2/2(Out2) -> Lower gear mesh/3, Mux/3  "K_A"
  From2/1 -> To Workspace5/1, Lower gear mesh/1  "RPM"
  From1/1 -> To Workspace2/1, Subsystem2/1(In3)
  From7/1 -> Max torque EC/1
  From8/1 -> MAX K_A EC/1
  From12/1 -> Max torque LG/1
  From11/1 -> MAX K_A LG/1
  Flex coupling rpm/1(vel) -> Goto/1  "RPM flex coupling"
  ? -> Goto2/1  "Torque gear mesh"
  Mux/1 -> T_rel/1
  ? -> Goto1/1  "Torque flex coupling"
  UGrpm/1(vel) -> Goto4/1  "RPM UG"
  Torque sensor1/1(signal) -> Goto5/1  "Torque UG"
  Subsystem1/1(Out1) -> Upper gear mesh/2  "T"
  Subsystem1/2(Out2) -> Upper gear mesh/3, Mux/2  "K_A"
  From10/1 -> To Workspace4/1, Upper gear mesh/1  "RPM"
  From3/1 -> To Workspace1/1, Subsystem1/1(In3)
  From9/1 -> Max torque UG/1
  From4/1 -> MAX K_A UG/1
  From5/1 -> Subsystem/1(T_in), To Workspace/1
  UGrpm/2(angle) -> To Workspace6/1
  Flex coupling rpm/2(angle) -> To Workspace8/1
  rpm2/2(angle) -> To Workspace9/1
  rpm1/2(angle) -> To Workspace10/1
  rpm3/2(angle) -> To Workspace11/1
  [Torque12] -> Mux3/12
  [Torque11] -> Mux3/11
  [AngularSpeed13] -> Mux1/13
  [AngularSpeed12] -> Mux1/12
  Mux3/1 -> Scope3/1, To Workspace14/1
  [Torque1] -> Mux3/1
  [Angle1] -> Mux2/1
  [AngularSpeed3] -> Mux1/3
  [AngularSpeed5] -> Mux1/5
  [Torque4] -> Mux3/4
  [AngularSpeed11] -> Mux1/11
  Clock/1 -> To Workspace15/1
  Mux2/1 -> Scope2/1, To Workspace13/1
  [Torque3] -> Mux3/3
  [Torque6] -> Mux3/6
  [AngularSpeed6] -> Mux1/6
  [AngularSpeed1] -> Mux1/1
  [Angle3] -> Mux2/3
  [TorqueMotor] -> Scope4/1, To Workspace16/1
  [Torque5] -> Mux3/5
  [AngularSpeed2] -> Mux1/2
  [Torque8] -> Mux3/8
  [Angle2] -> Mux2/2
  [AngularSpeed8] -> Mux1/8
  [AngularSpeed10] -> Mux1/10
  [Torque10] -> Mux3/10
  [AngularSpeed9] -> Mux1/9
  [Torque2] -> Mux3/2
  Mux1/1 -> Scope1/1, To Workspace12/1
  [Torque7] -> Mux3/7
  [Torque9] -> Mux3/9
  [AngularSpeed7] -> Mux1/7
  [AngularSpeed4] -> Mux1/4
  [AngularSpeed22] -> Mux1/22
  [AngularSpeed21] -> Mux1/21
  [AngularSpeed20] -> Mux1/20
  [AngularSpeed19] -> Mux1/19
  [AngularSpeed18] -> Mux1/18
  [AngularSpeed17] -> Mux1/17
  [AngularSpeed16] -> Mux1/16
  [AngularSpeed15] -> Mux1/15
  [AngularSpeed14] -> Mux1/14
  [Angle4] -> Mux2/4
  [Angle5] -> Mux2/5
  [Angle6] -> Mux2/6
  [Angle7] -> Mux2/7
  [Angle8] -> Mux2/8
  [Angle9] -> Mux2/9
  [Angle10] -> Mux2/10
  [Angle11] -> Mux2/11
  [Angle12] -> Mux2/12
  [Angle13] -> Mux2/13
  [Angle22] -> Mux2/22
  [Angle21] -> Mux2/21
  [Angle20] -> Mux2/20
  [Angle19] -> Mux2/19
  [Angle18] -> Mux2/18
  [Angle17] -> Mux2/17
  [Angle16] -> Mux2/16
  [Angle15] -> Mux2/15
  [Angle14] -> Mux2/14
  [Torque13] -> Mux3/13
  [Torque14] -> Mux3/14
  [Torque15] -> Mux3/15
  [Torque16] -> Mux3/16
  [Torque17] -> Mux3/17
  [Torque18] -> Mux3/18
  [Torque19] -> Mux3/19
  [Torque20] -> Mux3/20
  [Torque21] -> Mux3/21
  [TorquePropeller] -> Scope4/2, To Workspace17/1
  connections:
  Signals 20/RConn1 -- C8/LConn1 -- K8/LConn1
  Signals 14/LConn1 -- "I5, Gear coupling"/LConn1 -- K5-6/RConn1 -- C5-6/RConn1
  Signals 15/LConn1 -- "I4, Gear coupling"/LConn1 -- K4_5/RConn1 -- C4_5/RConn1
  K9/LConn1 -- C9/LConn1 -- Signals 9/RConn1
  Signals 10/LConn1 -- Upper pinion2/LConn1 -- C9/RConn1 -- K9/RConn1
  K3-1/RConn1 -- C3-1/RConn1 -- "I4, Gear coupling2"/LConn1 -- Pinion/LConn1 -- LG/LConn1
  C5/LConn1 -- Signals 11/RConn1 -- K5/LConn1
  K3-1/LConn1 -- Signals 16/RConn1 -- C3-1/LConn1
  K4/RConn1 -- C4/RConn1 -- Signals 18/LConn1 -- Upper pinion5/LConn1
  Upper pinion6/LConn1 -- K6/RConn1 -- C6/RConn1 -- Signals 19/LConn1
  Propeller2/LConn1 -- Upper pinion9/LConn1 -- K10/RConn1 -- C10/RConn1 -- Prop shaft rpm/LConn1
  Upper pinion8/LConn1 -- Signals 21/LConn1 -- C8/RConn1 -- K8/RConn1
  C5/RConn1 -- UG/LConn1 -- Upper pinion14/LConn1 -- Upper pinion10/LConn1 -- K5/RConn1
  K13/RConn1 -- C13/RConn1 -- Signals 6/LConn1 -- Upper pinion16/LConn1
  K14/RConn1 -- Signals 4/LConn1 -- Upper pinion15/LConn1 -- C14/RConn1
  Upper pinion11/LConn1 -- Signals 5/LConn1 -- C12/RConn1 -- K12/RConn1
  K11/RConn1 -- Signals 7/LConn1 -- Upper pinion12/LConn1 -- C11/RConn1
  Signals 8/LConn1 -- Upper pinion19/LConn1 -- C15/RConn1 -- K15/RConn1
  Upper pinion1/LConn1 -- Signals Motor/RConn1 -- Signals 1/LConn1
  K17/RConn1 -- Signals 2/LConn1 -- Upper pinion13/LConn1 -- C17/RConn1
  UG/RConn1 -- Upper pinion18/LConn1 -- Signals 12/LConn1
  C3/RConn1 -- Signals 13/LConn1 -- Upper wheel/LConn1 -- K3/RConn1
  C4/LConn1 -- K4/LConn1 -- Signals 17 gear/RConn1
  electric motor/LConn1 -- Signals Motor/LConn1
  C14/LConn1 -- Signals 3/RConn1 -- K14/LConn1
  C12/LConn1 -- Signals 4/RConn1 -- K12/LConn1
  K13/LConn1 -- Signals 5/RConn1 -- C13/LConn1
  C11/LConn1 -- Signals 6/RConn1 -- K11/LConn1
  K15/LConn1 -- C15/LConn1 -- Signals 7/RConn1
  Signals 8/RConn1 -- C2/LConn1 -- K2/LConn1
  C2/RConn1 -- Upper pinion4/LConn1 -- Signals 9/LConn1 -- K2/RConn1
  K1/LConn1 -- C1/LConn1 -- Signals 10/RConn1
  Upper pinion3/LConn1 -- Signals 11/LConn1 -- C1/RConn1 -- K1/RConn1
  Signals 12/RConn1 -- K3/LConn1 -- C3/LConn1
  C5-6/LConn1 -- Signals 13/RConn1 -- K5-6/LConn1
  C4_5/LConn1 -- K4_5/LConn1 -- Signals 14/RConn1
  C3-4/LConn1 -- Signals 15/RConn1 -- K3-4/LConn1
  K3-4/RConn1 -- "I4, Gear coupling1"/LConn1 -- Signals 16/LConn1 -- C3-4/RConn1
  Signals 17 gear/LConn1 -- Pinion1/LConn1 -- LG/RConn1
  K6/LConn1 -- C6/LConn1 -- Signals 18/RConn1
  K7/LConn1 -- C7/LConn1 -- Signals 19/RConn1
  C7/RConn1 -- Upper pinion7/LConn1 -- Signals 20/LConn1 -- K7/RConn1
  C10/LConn1 -- K10/LConn1 -- Signals 21/RConn1
  Signals 1/RConn1 -- K17/LConn1 -- C17/LConn1
  Signals 2/RConn1 -- K16/LConn1 -- C16/LConn1
  K16/RConn1 -- C16/RConn1 -- Upper pinion17/LConn1 -- Signals 3/LConn1
